simulink model "mpcSetpointIpopt"  (Simulink 7.9)
settings: Solver=ode4  StartTime=0.0  StopTime=200  RelTol=1e-3
values from neighbouring files (symbols this model uses):
  A = params.A    [cvxsolve.m]    (also in prepSoftFewerSlacks.m = [1 dt 0.5*dt*dt; prepSoftKS.m = [1 dt 0.5*dt*dt; prepSoftKS_coupled.m = [1 dt 0.5*dt*dt; prepSoftQuadprog.m = [1 dt 0.5*dt*dt)
  B = params.B    [cvxsolve.m]    (also in prepSoftFewerSlacks.m = B*[1 0]; prepSoftKS.m = [0.5*dt*dt; prepSoftKS_coupled.m = [0.5*dt*dt; prepSoftQuadprog.m = B*[1 0])
  bd = [kron(ones(T,1),eye(n))]    [prepSoftFewerSlacks.m]    (also in prepSoftKS.m = [kron(ones(T,1),eye(n)); -Ed]; prepSoftKS_coupled.m = [kron(ones(T,1),eye(n)); [1 0 0; 0 1 0]]; prepSoftQuadprog.m)
  bx = [A; zeros(ellef+(T-1)*n,n)]    [prepSoftFewerSlacks.m]    (also in prepSoftKS.m; prepSoftKS_coupled.m; prepSoftQuadprog.m)
  C = [kron(eye(T),[-B eye(n)]) + kron([zeros(1,T); eye(T-1) zeros(T-1,1)],[zeros(n,m) -A]); zeros(ellef,m+(T-1)*(m+n)) Ef]    [prepSoftFewerSlacks.m]    (also in prepSoftKS.m; prepSoftKS_coupled.m; prepSoftQuadprog.m)
  dt = 0.25    [prepSoftFewerSlacks.m]    (also in prepSoftKS.m; prepSoftKS_coupled.m; prepSoftQuadprog.m)
  Ff = params.Ff    [cvxsolve.m]    (also in prepSoftFewerSlacks.m = [0 0 1; prepSoftKS.m = 0.00001*[eye(2) [0;0]; -eye(2) [0;0]]; prepSoftKS_coupled.m = 0.00001*[eye(2) [0;0]; -eye(2) [0;0]]; prepSoftQuadprog.m = [0 0 1)
  Fu = params.Fu    [cvxsolve.m]    (also in prepSoftFewerSlacks.m = [Fu*[1 0]; Fus (0*fs - 1); [0 -1] ]; prepSoftKS.m = [1; prepSoftKS_coupled.m = [0; prepSoftQuadprog.m = [Fu*[1 0]; Fus (0*fs - 1); [0 -1] ])
  Fus = params.Fus    [cvxsolve.m]    (also in prepSoftFewerSlacks.m = Fus*[1 0]; prepSoftKS.m = [0; prepSoftKS_coupled.m = [0; prepSoftQuadprog.m = Fus*[1 0])
  Fx = params.Fx    [cvxsolve.m]    (also in prepSoftFewerSlacks.m = [Fx;Fxs;zeros(1,size(A,1))]; prepSoftKS.m = [0 0 0; prepSoftKS_coupled.m = [0 0 1; prepSoftQuadprog.m = [Fx;Fxs;zeros(1,size(A,1))])
  Fxs = params.Fxs    [cvxsolve.m]    (also in prepSoftFewerSlacks.m = [0 1 0; prepSoftKS.m = [0 1 0; prepSoftKS_coupled.m = [0.1 1 0; prepSoftQuadprog.m = [0 1 0)
  g = [r; repmat([q;r],T-1,1); qf]    [prepSoftFewerSlacks.m]    (also in prepSoftKS.m; prepSoftKS_coupled.m; prepSoftQuadprog.m)
  gt = kron(ones(T,1),[zeros(2,n); -2*Q])    [prepSoftFewerSlacks.m]    (also in prepSoftKS.m = kron(ones(T,1),[zeros(1,n); -2*Q]); prepSoftKS_coupled.m = kron(ones(T,1),[zeros(1,n); -2*Q]); prepSoftQuadprog.m)
  H = blkdiag(R,kron(eye(T-1),blkdiag(Q,R)),Qf)    [prepSoftFewerSlacks.m]    (also in prepSoftKS.m; prepSoftKS_coupled.m; prepSoftQuadprog.m)
  hc = [repmat(f,T,1);ff]    [prepSoftFewerSlacks.m]    (also in prepSoftKS.m; prepSoftKS_coupled.m; prepSoftQuadprog.m)
  hcs = [repmat(fs,T,1)]    [prepSoftFewerSlacks.m]    (also in prepSoftKS.m; prepSoftKS_coupled.m; prepSoftQuadprog.m)
  hx = [-Fx; zeros((T-1)*ell + ellf,n)]    [prepSoftFewerSlacks.m]    (also in prepSoftKS.m; prepSoftKS_coupled.m; prepSoftQuadprog.m)
  hxs = [-Fxs; zeros((T-1)*ells,n)]    [prepSoftFewerSlacks.m]    (also in prepSoftKS.m; prepSoftKS_coupled.m; prepSoftQuadprog.m)
  m = size(B,2)    [ipoptSolve.m]    (also in ipoptSolve2.m; mpcsolve.m; mpcsolve_ipopt.m; prepSoftFewerSlacks.m)
  n = size(A,1)    [ipoptSolve.m]    (also in ipoptSolve2.m; mpcsolve.m = size(AT,1)/2; mpcsolve_ipopt.m; prepSoftFewerSlacks.m)
  opts = []    [prepSoftKS.m]    (also in prepSoftKS_coupled.m)
  P = blkdiag(Fu,kron(eye(T-1),[Fx Fu]),Ff)    [prepSoftFewerSlacks.m]    (also in prepSoftKS.m; prepSoftKS_coupled.m; prepSoftQuadprog.m)
  Ps = blkdiag(Fus,kron(eye(T-1),[Fxs Fus]))    [prepSoftFewerSlacks.m]    (also in prepSoftKS.m; prepSoftKS_coupled.m; prepSoftQuadprog.m)
  Q = params.Q    [cvxsolve.m]    (also in prepSoftFewerSlacks.m = diag([5 5 2]); prepSoftKS.m = diag([5 5 2]); prepSoftKS_coupled.m = diag([5 5 2]); prepSoftQuadprog.m = diag([5 5 2]))
  Qf = Q    [prepSoftFewerSlacks.m]    (also in prepSoftKS.m = diag([5 5 2]); prepSoftKS_coupled.m = diag([5 5 2]); prepSoftQuadprog.m = diag([5 5 2]))
  R = params.R    [cvxsolve.m]    (also in prepSoftFewerSlacks.m = blkdiag(R, 0.00001); prepSoftKS.m = diag([10]); prepSoftKS_coupled.m = diag([10]); prepSoftQuadprog.m = blkdiag(R, 0.00001))
  T = linsolve(cholM,eye(size(M,1)),struct('LT',true))    [ipoptSolve.m]    (also in ipoptSolve2.m; mpcsolve.m = (ne-ellef)/size(A,1); mpcsolve_ipopt.m; prepSoftFewerSlacks.m = 10)
undefined symbols (not defined in the file or in its folder): Ef_block
libraries: simulink x1
settings Model: Creator=aeagr  LastModifiedBy=aeagr
settings DebuggingCC: StrictBusMsg=Warning
settings GRTTargetCC: CombineOutputUpdateFcns=off  GRTInterface=on

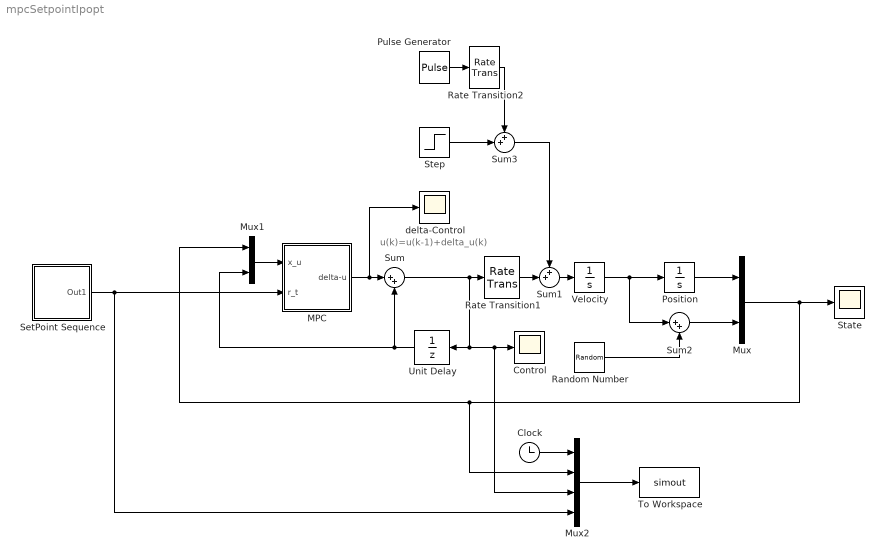
== system mpcSetpointIpopt ==
  note: u(k)=u(k-1)+delta_u(k)
  Clock : Clock
  Control : Scope
      settings: TimeRange=240  YMin=-0.4  YMax=0.35
  MPC : Subsystem  RequirementInfo="{}  %GIDa_0c6e92d2_bf34_4970_87ae_4e32833bf9c6"  TreatAsAtomicUnit=on  SystemSampleTime=dt
      settings: RTWSystemCode=Function  RTWFcnNameOpts=Use subsystem name  RTWFileNameOpts=Use subsystem name
  Mux : Mux  Inputs=2
  Mux1 : Mux  Inputs=2
  Mux2 : Mux
  Position : Integrator
  Pulse Generator : DiscretePulseGenerator  PulseType=Time based  Amplitude=0.1  Period=200  PhaseDelay=100
  Random Number : RandomNumber  Variance=0.000000001  SampleTime=dt
  Rate Transition1 : RateTransition
  Rate Transition2 : RateTransition
  SetPoint Sequence : Subsystem
  State : Scope
      settings: TimeRange=200  YMin=-1  YMax=14
  Step : Step  Time=100  After=0.01  SampleTime=0
  Sum : Sum  Inputs=|++
  Sum1 : Sum  Inputs=++|
  Sum2 : Sum  Inputs=|++
  Sum3 : Sum  Inputs=++|
  To Workspace : ToWorkspace  VariableName=simout  SampleTime=-1
  Unit Delay : UnitDelay  SampleTime=dt
  Velocity : Integrator
  delta-Control : Scope
      settings: TimeRange=240  YMin=-0.4  YMax=0.35  SaveName=ScopeData2
  wires:
  Velocity/1 -> Position/1, Sum2/1
  Mux/1 -> State/1, Mux2/2, Mux1/1
  Position/1 -> Mux/1
  SetPoint Sequence/1(Out1) -> Mux2/4, MPC/2(r_t)
  Sum/1 -> Unit Delay/1, Control/1, Mux2/3, Rate Transition1/1
  Unit Delay/1 -> Sum/2, Mux1/2
  MPC/1(delta-u) -> Sum/1, delta-Control/1
  Mux1/1 -> MPC/1(x_u)
  Sum1/1 -> Velocity/1
  Mux2/1 -> To Workspace/1
  Clock/1 -> Mux2/1
  Sum2/1 -> Mux/2
  Random Number/1 -> Sum2/2
  Rate Transition1/1 -> Sum1/2
  Step/1 -> Sum3/2
  Sum3/1 -> Sum1/1
  Pulse Generator/1 -> Rate Transition2/1
  Rate Transition2/1 -> Sum3/1

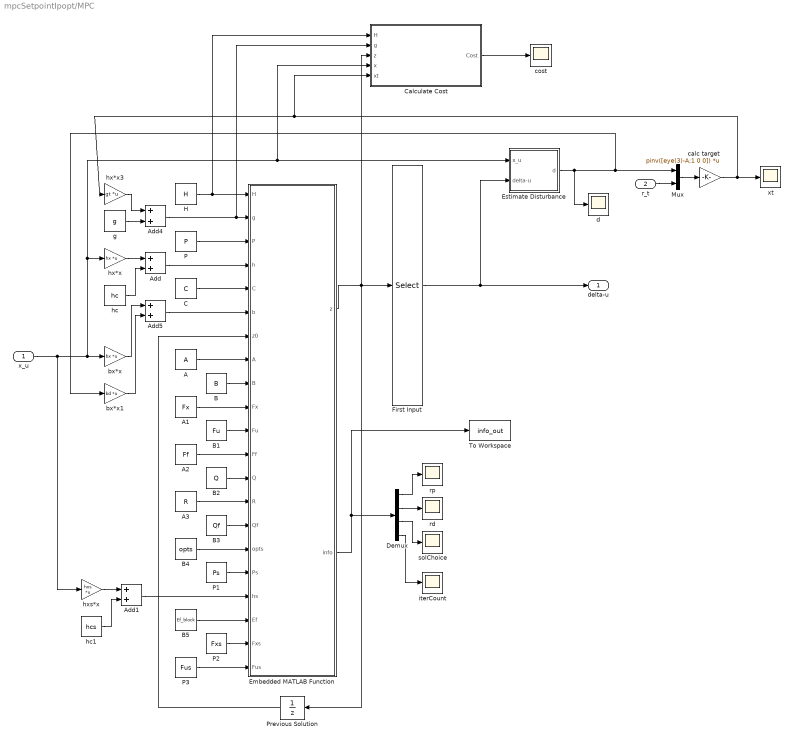
== system mpcSetpointIpopt/MPC ==
  x_u : Inport
  r_t : Inport  Port=2
  A : Constant  Value=A
  A1 : Constant  Value=Fx
  A2 : Constant  Value=Ff
  A3 : Constant  Value=R
  Add{,1,4..5} (4 alike) : Sum
  B : Constant  Value=B
  B1 : Constant  Value=Fu
  B2 : Constant  Value=Q
  B3 : Constant  Value=Qf
  B4 : Constant  Value=opts
  B5 : Constant  Value=Ef_block
  C : Constant  Value=C
  Calculate Cost : Subsystem
  Demux : Demux
  Embedded MATLAB Function : MATLAB Function  TreatAsAtomicUnit=on
      settings: RTWFileNameOpts=Use subsystem name
  Estimate Disturbance : Subsystem
  First Input : Selector  InputPortWidth=T*(n+m)  IndexOptions=Index vector (dialog)  Indices=1  OutputSizes=1
  H : Constant  Value=H
  Mux : Mux  Inputs=2
  P : Constant  Value=P
  P1 : Constant  Value=Ps
  P2 : Constant  Value=Fxs
  P3 : Constant  Value=Fus
  Previous Solution : UnitDelay  SampleTime=-1
  To Workspace : ToWorkspace  VariableName=info_out  SampleTime=-1
  bx*x : Gain  Gain=bx  Multiplication=Matrix(K*u)
  bx*x1 : Gain  Gain=bd  Multiplication=Matrix(K*u)
  calc target : Gain  Gain=pinv([eye(3)-A;1 0 0])  Multiplication=Matrix(K*u)
  cost : Scope
      settings: YMin=-0.25  YMax=2.5  SaveName=ScopeData8
  d : Scope
      settings: YMin=-0.00025  YMax=0.002  SaveName=ScopeData6
  g : Constant  Value=g
  hc : Constant  Value=hc
  hc1 : Constant  Value=hcs
  hx*x : Gain  Gain=hx  Multiplication=Matrix(K*u)
  hx*x3 : Gain  Gain=gt  Multiplication=Matrix(K*u)
  hxs*x : Gain  Gain=hxs  Multiplication=Matrix(K*u)
  iterCount : Scope
      settings: TimeRange=200  YMin=0  YMax=25  SaveName=ScopeData9
  rd : Scope
      settings: YMin=0  YMax=13  SaveName=ScopeData4
  rp : Scope
      settings: YMin=1.65436e-24  YMax=2.75e-08  SaveName=ScopeData3
  solChoice : Scope
      settings: YMin=0.95  YMax=1.05  SaveName=ScopeData5
  xt : Scope
      settings: YMin=-0.25  YMax=2.5  SaveName=ScopeData7
  delta-u : Outport
  wires:
  First Input/1 -> delta-u/1, Estimate Disturbance/2(delta-u)
  Embedded MATLAB Function/1(z) -> Previous Solution/1, First Input/1, Calculate Cost/3(z)
  Previous Solution/1 -> Embedded MATLAB Function/7(z0)
  H/1 -> Embedded MATLAB Function/1(H), Calculate Cost/1(H)
  P/1 -> Embedded MATLAB Function/3(P)
  C/1 -> Embedded MATLAB Function/5(C)
  Add/1 -> Embedded MATLAB Function/4(h)
  x_u/1 -> bx*x/1, hx*x/1, Estimate Disturbance/1(x_u), Calculate Cost/4(x), hxs*x/1
  hx*x/1 -> Add/1
  hc/1 -> Add/2
  B/1 -> Embedded MATLAB Function/9(B)
  A/1 -> Embedded MATLAB Function/8(A)
  B3/1 -> Embedded MATLAB Function/15(Qf)
  A3/1 -> Embedded MATLAB Function/14(R)
  B2/1 -> Embedded MATLAB Function/13(Q)
  A2/1 -> Embedded MATLAB Function/12(Ff)
  B1/1 -> Embedded MATLAB Function/11(Fu)
  A1/1 -> Embedded MATLAB Function/10(Fx)
  Embedded MATLAB Function/2(info) -> Demux/1, To Workspace/1
  Demux/1 -> rp/1
  Demux/2 -> rd/1
  Demux/3 -> solChoice/1
  B4/1 -> Embedded MATLAB Function/16(opts)
  P1/1 -> Embedded MATLAB Function/17(Ps)
  hxs*x/1 -> Add1/1
  hc1/1 -> Add1/2
  Add1/1 -> Embedded MATLAB Function/18(hs)
  Estimate Disturbance/1(d) -> Mux/1, bx*x1/1, d/1
  Mux/1 -> calc target/1
  r_t/1 -> Mux/2
  calc target/1 -> xt/1, hx*x3/1, Calculate Cost/5(xt)
  Add4/1 -> Embedded MATLAB Function/2(g), Calculate Cost/2(g)
  g/1 -> Add4/2
  hx*x3/1 -> Add4/1
  Add5/1 -> Embedded MATLAB Function/6(b)
  bx*x/1 -> Add5/1
  bx*x1/1 -> Add5/2
  B5/1 -> Embedded MATLAB Function/19(Ef)
  P2/1 -> Embedded MATLAB Function/20(Fxs)
  P3/1 -> Embedded MATLAB Function/21(Fus)
  Calculate Cost/1(Cost) -> cost/1
  Demux/4 -> iterCount/1

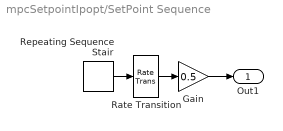
== system mpcSetpointIpopt/SetPoint Sequence ==
  Gain : Gain  Gain=0.5
  Rate Transition : RateTransition
  Repeating Sequence Stair : simulink/Sources/Repeating Sequence Stair  OutValues=[1 0 2 0 3 0 4 0 5 0 6 0].'  tsamp=20  OutMin=[]  OutMax=[]  OutDataTypeStr=double  OutputDataTypeScalingMode=Specify via dialog  OutDataType=double  ConRadixGroup=Best Precision: Vector-wise  OutScaling=2^-12
  Out1 : Outport
  wires:
  Repeating Sequence Stair/1 -> Rate Transition/1
  Rate Transition/1 -> Gain/1
  Gain/1 -> Out1/1

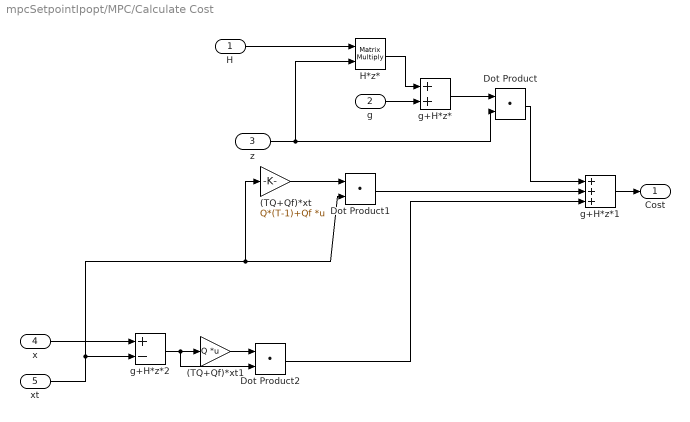
== system mpcSetpointIpopt/MPC/Calculate Cost ==
  H : Inport
  g : Inport  Port=2
  z : Inport  Port=3
  x : Inport  Port=4
  xt : Inport  Port=5
  (TQ+Qf)*xt : Gain  Gain=Q*(T-1)+Qf  Multiplication=Matrix(K*u)
  (TQ+Qf)*xt1 : Gain  Gain=Q  Multiplication=Matrix(K*u)
  Dot Product : DotProduct  InputSameDT=on  OutDataTypeStr=Inherit: Inherit via internal rule
  Dot Product1 : DotProduct  InputSameDT=on  OutDataTypeStr=Inherit: Inherit via internal rule
  Dot Product2 : DotProduct  InputSameDT=on  OutDataTypeStr=Inherit: Inherit via internal rule
  H*z* : Product  Multiplication=Matrix(*)  RndMeth=Zero
  g+H*z* : Sum
  g+H*z*1 : Sum  Inputs=+++
  g+H*z*2 : Sum  Inputs=+-
  Cost : Outport
  wires:
  H*z*/1 -> g+H*z*/1
  g+H*z*/1 -> Dot Product/1
  (TQ+Qf)*xt/1 -> Dot Product1/1
  Dot Product/1 -> g+H*z*1/1
  Dot Product1/1 -> g+H*z*1/2
  g+H*z*2/1 -> (TQ+Qf)*xt1/1, Dot Product2/2
  (TQ+Qf)*xt1/1 -> Dot Product2/1
  Dot Product2/1 -> g+H*z*1/3
  H/1 -> H*z*/1
  g/1 -> g+H*z*/2
  z/1 -> H*z*/2, Dot Product/2
  x/1 -> g+H*z*2/1
  xt/1 -> g+H*z*2/2, (TQ+Qf)*xt/1, Dot Product1/2
  g+H*z*1/1 -> Cost/1

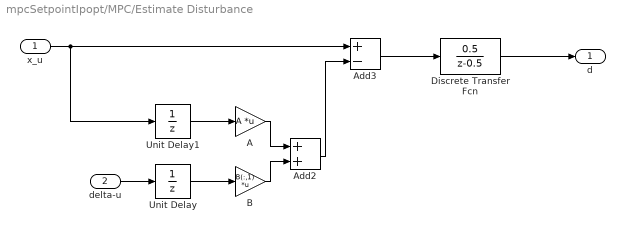
== system mpcSetpointIpopt/MPC/Estimate Disturbance ==
  x_u : Inport
  delta-u : Inport  Port=2
  A : Gain  Gain=A  Multiplication=Matrix(K*u)
  Add2 : Sum
  Add3 : Sum  Inputs=+-
  B : Gain  Gain=B(:,1)  Multiplication=Matrix(K*u)
  Discrete Transfer Fcn : DiscreteTransferFcn  Numerator=[0.5]  Denominator=[1 -0.5]
  Unit Delay : UnitDelay  SampleTime=-1
  Unit Delay1 : UnitDelay  SampleTime=-1
  d : Outport
  wires:
  Unit Delay1/1 -> A/1
  Unit Delay/1 -> B/1
  A/1 -> Add2/1
  B/1 -> Add2/2
  Add2/1 -> Add3/2
  x_u/1 -> Unit Delay1/1, Add3/1
  delta-u/1 -> Unit Delay/1
  Add3/1 -> Discrete Transfer Fcn/1
  Discrete Transfer Fcn/1 -> d/1

== matlab function MPC/Embedded MATLAB Function ==
  data: H input double; z output double; g input double; P input double; h input double; C input double; b input double size=T*n+ellef; z0 input double; A input double; B input double; Fx input double; Fu input double; Ff input double; Q input double; R input double; Qf input double; info output double; opts input double; Ps input double; hs input double; Ef input double; Fxs input double; Fus input double
function [z,info] = mpcsolve_simk(H,g,P,h,C,b,z0,A,B,Fx,Fu,Ff,Q,R,Qf,opts,Ps,hs,Ef,Fxs,Fus)
%#codegen
coder.extrinsic('ipoptSolve2')

z = zeros(40,1);
info = zeros(4,1);

% just call to the Matlab version
[z,info] = ipoptSolve2(H,g,P,h,C,b,z0,A,B,Fx,Fu,Ff,Q,R,Qf,opts,Ps,hs,Ef,Fxs,Fus);
